simulink model "autotunerPID"  (Simulink 10.0)
settings: Solver=ode45  StartTime=0.0  StopTime=1000  FixedStep=0.005  RelTol=1e-5  EnableMultiTasking=on
undefined symbols (not defined in the file): Abutter, Bbutter
settings Model: Creator=root  LastModifiedBy=bhisma
settings DataIOCC: LimitDataPoints=on  SignalLoggingSaveFormat=ModelDataLogs  SaveOutput=off  SaveTime=off  SignalLoggingName=sigsOut
settings OptimizationCC: LifeSpan=auto
settings DebuggingCC: SaveWithParameterizedLinksMsg=none  SignalResolutionControl=TryResolveAllWithWarning  MultiTaskDSMMsg=warning  MultiTaskCondExecSysMsg=none  SFUnexpectedBacktrackingDiag=error  SFNoUnconditionalDefaultTransitionDiag=error  SFExecutionAtInitializationDiag=warning  ArithmeticOperatorsInVariantConditions=error
settings HardwareCC: TargetUnknown=on
settings SFSimCC: SimUseLocalCustomCode=on  CustomCodeUndefinedFunction=FilterOut
settings RTWCC: RTWUseLocalCustomCode=on
settings CodeAppCC: StateflowObjectComments=off
settings GRTTargetCC: TargetLangStandard=C99 (ISO)

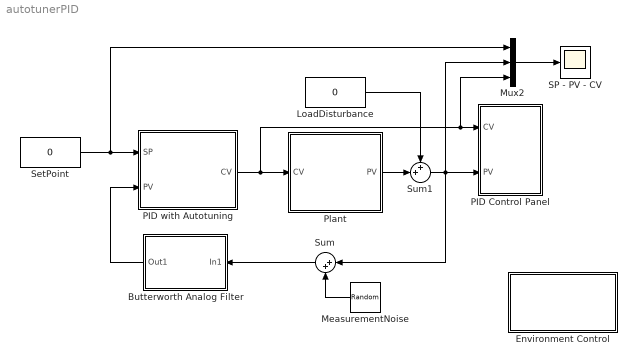
== system autotunerPID ==
  Butterworth Analog Filter : Subsystem  mask{Wc=100, N=2}
      mask prompts: Wc "Bandwidth (Wc)"; N "Filter order (N)"
      mask init:
      | [Bbutter,Abutter] = butterdesign(N,Wc);
      mask Display: disp('Butterworth\nFilter')
  Environment Control : Subsystem  StartFcn=|  StopFcn=|  mask(Pendulum plot){NoiseBlock=MeasurementNoise, LoadDistBlock=LoadDisturbance}
      StartFcn=|
      | global MODELRUNNING;
      | MODELRUNNING = 1;
      StopFcn=|
      | global MODELRUNNING;
      | MODELRUNNING = 0;
      mask prompts: NoiseBlock "Measurement noise signal block name"; LoadDistBlock "Load disturbance signal block"
      mask help: Pendulum plot
      mask Help: Pendulum animation function using Handle graphics.
      mask Display: disp('Environment\nControl')
  LoadDisturbance : Constant  Value=0
  MeasurementNoise : RandomNumber  Variance=0  SampleTime=0
  Mux2 : Mux  Inputs=3
  PID Control Panel : Subsystem  mask(Pendulum plot){RefBlock=SetPoint}
      mask prompts: RefBlock "Reference signal block name:"
      mask help: Pendulum plot
      mask Help: Pendulum animation function using Handle graphics.
      mask Display:
      | plot([-6 6 6 -6 -6],[-10 -10 10 10 -10])
      | patch([-5 -3 -3 -5],[4 4 -2 -2],[1 1 0])
      | plot([-5 -3 -3 -5 -5],[9 9 -2 -2 9])
      | patch([-1 1 1 -1],[2 2 -2 -2],[1 0 1])
      | plot([-1 1 1 -1 -1],[9 9 -2 -2 9])
      | patch([3 5 5 3],[7 7 -2 -2],[0 1 1])
      | plot([3 5 5 3 3],[9 9 -2 -2 9])
      | patch([-5 -2 -2 -5],[-4 -4 -6 -6],[0.4 0.4 0.4])
      | plot([-5 -2 -2 -5 -5],[-4 -4 -6 -6 -4])
      | patch([-5 2 2 -5],[-7 -7 -9 -9],[0.6 0.6 0.6])
      | plot([-5 2 2 -5 -5],[-7 -7 -9 -9 -7])
  PID with Autotuning : Subsystem  mask{K=1, Ti=2, Td=0.5, N=10, b=1, uaw=[-5 5], Ts=0.1, As=1, hystLevel=0.05}
      mask prompts: K "Gain (K)"; Ti "Integral time (Ti)"; Td "Derivative time (Td)"; N "Derivative Filter (N)"; b "Setpoint weigthing (b)"; uaw "Antiwindup saturation ([umin,umax])"; Ts "Sample time (Ts)"; As "Amplitude of the identifcation step or relay (As)"; hystLevel "Hysteresis of the relay (hystLevel)"
      mask init:
      | umin = uaw(1);
      | umax = uaw(2);
      | global PIDPARAMETERS;
      | PIDPARAMETERS = [K Ti Td N b];
      mask Display: disp('PID with\nAutotuning')
  Plant : Subsystem
      mask Display: disp('PLANT')
  SP - PV - CV : Scope
  SetPoint : Constant  Value=0
  Sum : Sum  Inputs=|++  SaturateOnIntegerOverflow=on  InputSameDT=on  OutDataTypeStr=Inherit: Same as first input
  Sum1 : Sum  Inputs=++|  SaturateOnIntegerOverflow=on  InputSameDT=on  OutDataTypeStr=Inherit: Same as first input
  wires:
  SetPoint/1 -> PID with Autotuning/1(SP), Mux2/1
  PID with Autotuning/1(CV) -> Plant/1(CV), PID Control Panel/1(CV), Mux2/3
  Mux2/1 -> SP - PV - CV/1
  MeasurementNoise/1 -> Sum/2
  Sum/1 -> Butterworth Analog Filter/1(In1)
  Plant/1(PV) -> Sum1/2
  Sum1/1 -> PID Control Panel/2(PV), Sum/1, Mux2/2
  LoadDisturbance/1 -> Sum1/1
  Butterworth Analog Filter/1(Out1) -> PID with Autotuning/2(PV)

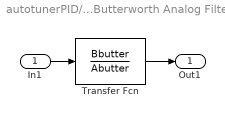
== system autotunerPID/Butterworth Analog Filter ==
  In1 : Inport
  Transfer Fcn : TransferFcn  Numerator=Bbutter  Denominator=Abutter
  Out1 : Outport
  wires:
  In1/1 -> Transfer Fcn/1
  Transfer Fcn/1 -> Out1/1

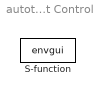
== system autotunerPID/Environment Control ==
  S-function : S-Function  FunctionName=envgui  Parameters=NoiseBlock,LoadDistBlock  SFunctionDeploymentMode=off  EnableBusSupport=off
      settings: DeleteFcn=pendan([],[],[],'DeleteBlock');

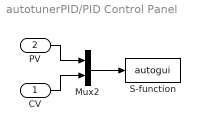
== system autotunerPID/PID Control Panel ==
  CV : Inport
  PV : Inport  Port=2
  Mux2 : Mux  Inputs=2
  S-function : S-Function  FunctionName=autogui  Parameters=RefBlock  SFunctionDeploymentMode=off  EnableBusSupport=off
      settings: DeleteFcn=pendan([],[],[],'DeleteBlock');
  wires:
  Mux2/1 -> S-function/1
  PV/1 -> Mux2/1
  CV/1 -> Mux2/2

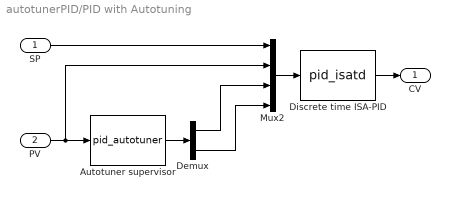
== system autotunerPID/PID with Autotuning ==
  SP : Inport
  PV : Inport  Port=2
  Autotuner supervisor : S-Function  FunctionName=pid_autotuner  Parameters=Ts,As  SFunctionDeploymentMode=off  EnableBusSupport=off
  Demux : Demux  Outputs=2
  Discrete time ISA-PID : S-Function  FunctionName=pid_isatd  Parameters=Ts,umin,umax,As,hystLevel  SFunctionDeploymentMode=off  EnableBusSupport=off
  Mux2 : Mux
  CV : Outport
  wires:
  Autotuner supervisor/1 -> Demux/1
  SP/1 -> Mux2/1
  PV/1 -> Mux2/2, Autotuner supervisor/1
  Discrete time ISA-PID/1 -> CV/1
  Mux2/1 -> Discrete time ISA-PID/1
  Demux/1 -> Mux2/3
  Demux/2 -> Mux2/4

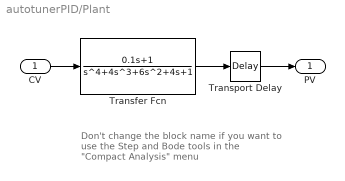
== system autotunerPID/Plant ==
  note: Don't change the block name
      | if you want to use the Step and Bode
      | tools in the "Compact Analysis" menu
  CV : Inport
  Transfer Fcn : TransferFcn  Numerator=[0.1 1]  Denominator=[1 4 6 4 1]
  Transport Delay : TransportDelay  DelayTime=0.75
  PV : Outport
  wires:
  Transfer Fcn/1 -> Transport Delay/1
  CV/1 -> Transfer Fcn/1
  Transport Delay/1 -> PV/1
